simulink model "Control_Validacao"  (R2015a)
settings: Solver=ode45  StartTime=0.0  StopTime=t(end)  RelTol=1e-3
values from neighbouring files (symbols this model uses):
  Cz = tf( [ 0.06455 -0.03577 0.005091 ] , [ 1 -0.6037 -0.3963 ] , T )    [Ident_RLtool.m]
  T = 0.04    [Ident_RLtool.m]
  Y1 = tf( [3.48e-6 1.6 6.079], [1 -0.2635 0.007111 0.009379], T )    [Ident_RLtool.m]
  Y2 = tf( [0.0003065 2.198 5.651], [1 -0.3892 0.1132 -0.03574], T )    [Ident_RLtool.m]
  Y3 = tf( [-1.216e-06 2.3 6.046], [1 -0.2409 -0.004502 0.01131], T )    [Ident_RLtool.m]
settings Model: Creator=Lucas  LastModifiedBy=Lucas

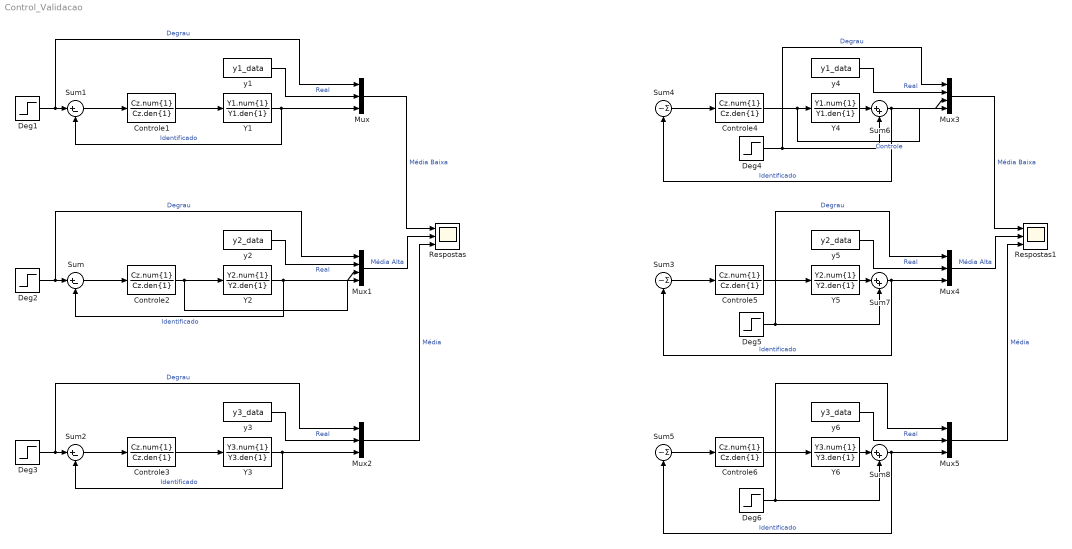
== system Control_Validacao ==
  Controle{1..6} (6 alike) : DiscreteTransferFcn  Numerator=Cz.num{1}  Denominator=Cz.den{1}  SampleTime=T
  Deg1 : Step  Time=5*T  After=100  SampleTime=T
  Deg2 : Step  Time=5*T  After=100  SampleTime=T
  Deg3 : Step  Time=5*T  After=100  SampleTime=T
  Deg4 : Step  Time=6*T  After=40  SampleTime=T
  Deg5 : Step  Time=6*T  After=40  SampleTime=T
  Deg6 : Step  Time=6*T  After=40  SampleTime=T
  Mux{,2,4..5} (4 alike) : Mux  Inputs=3
  Mux1 : Mux
  Mux3 : Mux
  Respostas : Scope  NumInputPorts=3
      settings: ShowLegends=on  TimeRange=1564  YMin=-5~-5~-5  YMax=5~5~5
  Respostas1 : Scope  NumInputPorts=3
      settings: ShowLegends=on  YMin=-5~-5~-5  YMax=5~5~5
  Sum : Sum  Inputs=|+-
  Sum1 : Sum  Inputs=|+-
  Sum2 : Sum  Inputs=|+-
  Sum3 : Sum  Inputs=|-
  Sum4 : Sum  Inputs=|-
  Sum5 : Sum  Inputs=|-
  Sum6 : Sum  Inputs=|++
  Sum7 : Sum  Inputs=|++
  Sum8 : Sum  Inputs=|++
  Y1 : DiscreteTransferFcn  Numerator=Y1.num{1}  Denominator=Y1.den{1}  SampleTime=T
  Y2 : DiscreteTransferFcn  Numerator=Y2.num{1}  Denominator=Y2.den{1}  SampleTime=T
  Y3 : DiscreteTransferFcn  Numerator=Y3.num{1}  Denominator=Y3.den{1}  SampleTime=T
  Y4 : DiscreteTransferFcn  Numerator=Y1.num{1}  Denominator=Y1.den{1}  SampleTime=T
  Y5 : DiscreteTransferFcn  Numerator=Y2.num{1}  Denominator=Y2.den{1}  SampleTime=T
  Y6 : DiscreteTransferFcn  Numerator=Y3.num{1}  Denominator=Y3.den{1}  SampleTime=T
  y1 : FromWorkspace  VariableName=y1_data  SampleTime=T
  y2 : FromWorkspace  VariableName=y2_data  SampleTime=T
  y3 : FromWorkspace  VariableName=y3_data  SampleTime=T
  y4 : FromWorkspace  VariableName=y1_data  SampleTime=T
  y5 : FromWorkspace  VariableName=y2_data  SampleTime=T
  y6 : FromWorkspace  VariableName=y3_data  SampleTime=T
  wires:
  Mux/1 -> Respostas/1  "Média Baixa"
  Y1/1 -> Sum1/2, Mux/3  "Identificado"
  Deg1/1 -> Sum1/1, Mux/1  "Degrau"
  y1/1 -> Mux/2  "Real"
  Y2/1 -> Sum/2, Mux1/3  "Identificado"
  Deg2/1 -> Mux1/1, Sum/1  "Degrau"
  y2/1 -> Mux1/2  "Real"
  Y3/1 -> Sum2/2, Mux2/3  "Identificado"
  Deg3/1 -> Sum2/1, Mux2/1  "Degrau"
  y3/1 -> Mux2/2  "Real"
  Mux2/1 -> Respostas/3  "Média"
  Mux1/1 -> Respostas/2  "Média Alta"
  Controle3/1 -> Y3/1
  Sum2/1 -> Controle3/1
  Controle2/1 -> Mux1/4, Y2/1
  Sum/1 -> Controle2/1
  Sum1/1 -> Controle1/1
  Controle1/1 -> Y1/1
  Mux3/1 -> Respostas1/1  "Média Baixa"
  Deg4/1 -> Sum6/2, Mux3/1  "Degrau"
  y4/1 -> Mux3/2  "Real"
  Deg5/1 -> Sum7/2, Mux4/1  "Degrau"
  y5/1 -> Mux4/2  "Real"
  Deg6/1 -> Sum8/2, Mux5/1
  y6/1 -> Mux5/2  "Real"
  Mux5/1 -> Respostas1/3  "Média"
  Mux4/1 -> Respostas1/2  "Média Alta"
  Controle6/1 -> Y6/1
  Sum5/1 -> Controle6/1
  Controle5/1 -> Y5/1
  Sum3/1 -> Controle5/1
  Sum4/1 -> Controle4/1
  Controle4/1 -> Mux3/4, Y4/1  "Controle"
  Y4/1 -> Sum6/1
  Sum6/1 -> Sum4/1, Mux3/3  "Identificado"
  Y5/1 -> Sum7/1
  Sum7/1 -> Sum3/1, Mux4/3  "Identificado"
  Y6/1 -> Sum8/1
  Sum8/1 -> Sum5/1, Mux5/3  "Identificado"
